simulink model "vehicle4"  (R2017a)
settings: Solver=VariableStepAuto  StartTime=0.0  StopTime=50  RelTol=1e-3
values from neighbouring files (symbols this model uses):
  Ts = 1    [dynorun.m]
undefined symbols (not defined in the file or in its folder): magnitude
undefined symbols (not defined in the file): containers
settings Model: Creator=tstef  LastModifiedBy=elts2

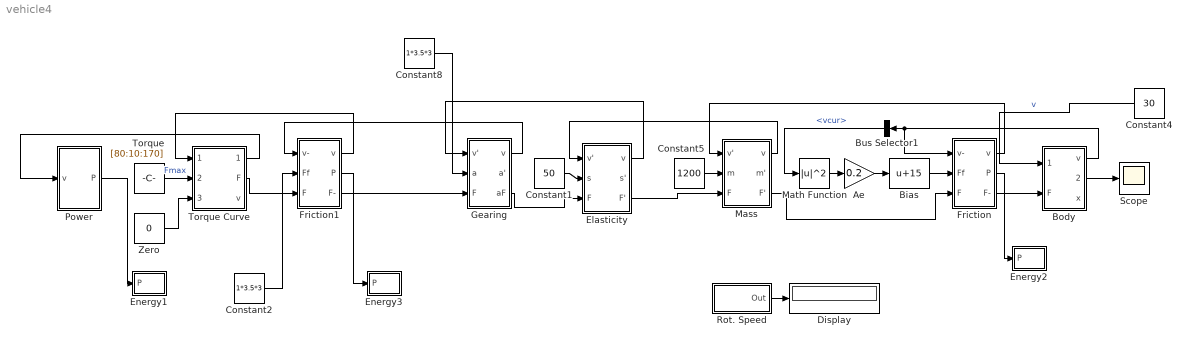
== system vehicle4 ==
  Ae : Gain  Gain=0.2
  Bias : Bias  Bias=15
  Body : Subsystem
  Bus Selector1 : BusSelector  OutputSignals=vcur
  Constant1 : Constant  Value=50
  Constant2 : Constant  Value=1*3.5*3
  Constant4 : Constant  Value=30
  Constant5 : Constant  Value=1200
  Constant8 : Constant  Value=1*3.5*3
  Display : Display
  Elasticity : Subsystem
  Energy1 : Subsystem
  Energy2 : Subsystem
  Energy3 : Subsystem
  Friction : Subsystem
  Friction1 : Subsystem
  Gearing : Subsystem
  Mass : Subsystem
  Math Function : Math  Operator=magnitude^2  SaturateOnIntegerOverflow=on
  Power : Subsystem
  Rot. Speed : Subsystem
  Scope : Scope
  Torque : Constant  Value=[80:10:170]
  Torque Curve : Subsystem
  Zero : Constant  Value=0
  wires:
  Constant8/1 -> Gearing/2(a)
  Gearing/3(aF) -> Elasticity/3(F)
  Mass/1(v) -> Elasticity/1(v')
  Mass/3(F') -> Friction/3(F)
  Friction/1(v) -> Mass/1(v')
  Constant5/1 -> Mass/2(m)
  Bias/1 -> Friction/2(Ff)
  Bus Selector1/1 -> Math Function/1  "<vcur>"
  Math Function/1 -> Ae/1
  Ae/1 -> Bias/1
  Gearing/1(v) -> Friction1/1(v-)
  Body/1(v) -> Bus Selector1/1, Friction/1(v-)
  Constant4/1 -> Body/1(vmax)  "v"
  Friction/3(F-) -> Body/2(F)
  Body/2(vcur) -> Scope/1
  Power/1(P) -> Energy1/1(P)
  Friction/2(P) -> Energy2/1(P)
  Elasticity/3(F') -> Mass/3(F)
  Elasticity/1(v) -> Gearing/1(v')
  Constant1/1 -> Elasticity/2(s)
  Rot. Speed/1(Out) -> Display/1
  Friction1/3(F-) -> Gearing/3(F)
  Friction1/1(v) -> Torque Curve/1(vreq)
  Constant2/1 -> Friction1/2(Ff)
  Friction1/2(P) -> Energy3/1(P)
  Torque Curve/2(F) -> Friction1/3(F)
  Torque Curve/1(vmax) -> Power/1(v)
  Torque/1 -> Torque Curve/2(Fmax)  "Fmax"
  Zero/1 -> Torque Curve/3(Fmin)

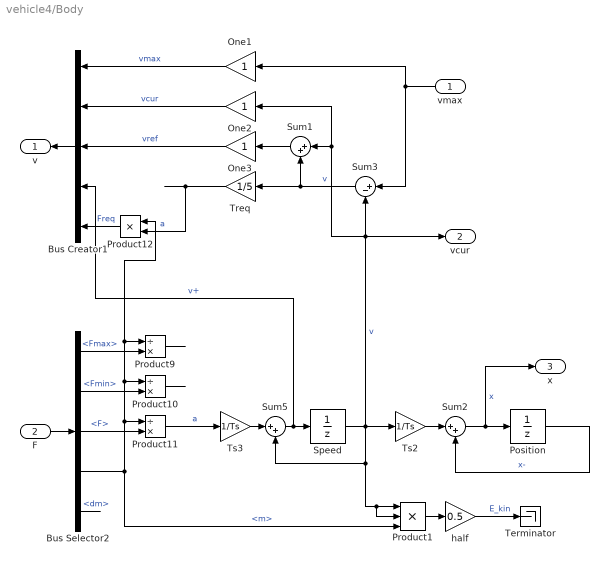
== system vehicle4/Body ==
  vmax : Inport  Unit=m/s
  F : Inport  Port=2
  Bus Creator1 : BusCreator  Inputs=5
  Bus Selector2 : BusSelector  OutputSignals=Fmax,Fmin,F,m,dm
  One1 : Gain
  One2 : Gain
  One3 : Gain
  Position : UnitDelay  InitialCondition=zeros(1,10)  SampleTime=Ts
  Product1 : Product  Inputs=***
  Product10 : Product  Inputs=/*
  Product11 : Product  Inputs=/*
  Product12 : Product
  Product9 : Product  Inputs=/*
  Speed : UnitDelay  InitialCondition=zeros(1,10)  SampleTime=Ts
  Sum1 : Sum  Inputs=|++
  Sum2 : Sum  Inputs=|++
  Sum3 : Sum  Inputs=|+-
  Sum5 : Sum  Inputs=|++
  Terminator : Terminator
  Treq : Gain  Gain=1/5
  Ts2 : Gain  Gain=1/Ts
  Ts3 : Gain  Gain=1/Ts
  half : Gain  Gain=0.5
  v : Outport
  vcur : Outport  Port=2
  x : Outport  Port=3
  wires:
  Treq/1 -> Product12/2  "a"
  Product11/1 -> Ts3/1  "a"
  One3/1 -> Bus Creator1/3  "vref"
  Product12/1 -> Bus Creator1/5  "Freq"
  Bus Selector2/5 -> ?  "<dm>"
  Sum1/1 -> One3/1
  One1/1 -> Bus Creator1/1  "vmax"
  F/1 -> Bus Selector2/1
  Bus Selector2/1 -> Product9/2  "<Fmax>"
  Bus Selector2/4 -> Product1/3, Product9/1, Product12/1, Product10/1, Product11/1  "<m>"
  Bus Selector2/3 -> Product11/2  "<F>"
  Bus Selector2/2 -> Product10/2  "<Fmin>"
  One2/1 -> Bus Creator1/2  "vcur"
  Speed/1 -> Ts2/1, vcur/1, Sum1/1, One2/1, Sum3/2, Sum5/2, Product1/2, Product1/1  "v"
  vmax/1 -> Sum3/1, One1/1
  Sum3/1 -> Sum1/2, Treq/1  "v"
  Sum5/1 -> Bus Creator1/4, Speed/1  "v+"
  Ts3/1 -> Sum5/1
  Product9/1 -> ?
  Product10/1 -> ?
  Bus Creator1/1 -> v/1
  Product1/1 -> half/1
  half/1 -> Terminator/1  "E_kin"
  Sum2/1 -> x/1, Position/1  "x"
  Position/1 -> Sum2/2  "x-"
  Ts2/1 -> Sum2/1

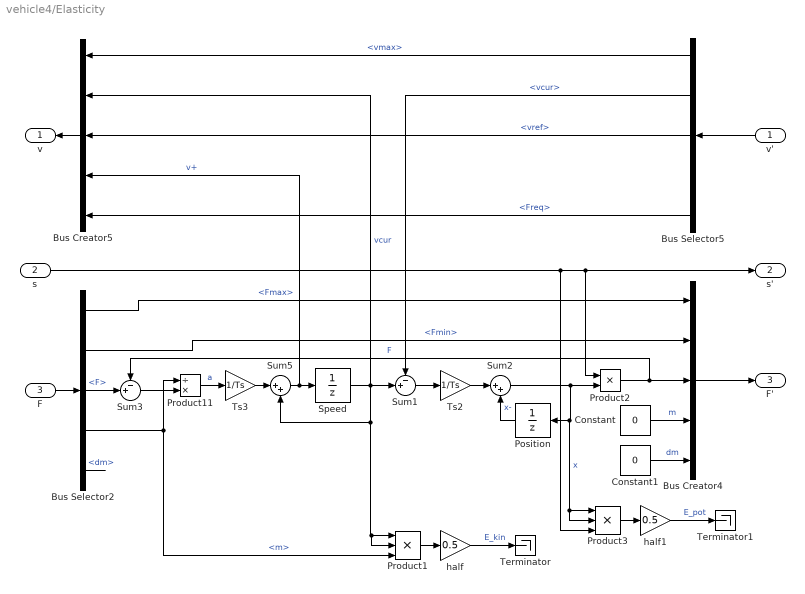
== system vehicle4/Elasticity ==
  v' : Inport
  s : Inport  Port=2
  F : Inport  Port=3
  Bus Creator4 : BusCreator  Inputs=5
  Bus Creator5 : BusCreator  Inputs=5
  Bus Selector2 : BusSelector  OutputSignals=Fmax,Fmin,F,m,dm
  Bus Selector5 : BusSelector  OutputSignals=vmax,vcur,vref,v+,Freq
  Constant : Constant  Value=0
  Constant1 : Constant  Value=0
  Position : UnitDelay  InitialCondition=zeros(1,10)  SampleTime=Ts
  Product1 : Product  Inputs=***
  Product11 : Product  Inputs=/*
  Product2 : Product  Inputs=**
  Product3 : Product  Inputs=***
  Speed : UnitDelay  InitialCondition=zeros(1,10)  SampleTime=Ts
  Sum1 : Sum  Inputs=-+|
  Sum2 : Sum  Inputs=|++
  Sum3 : Sum  Inputs=-+|
  Sum5 : Sum  Inputs=|++
  Terminator : Terminator
  Terminator1 : Terminator
  Ts2 : Gain  Gain=1/Ts
  Ts3 : Gain  Gain=1/Ts
  half : Gain  Gain=0.5
  half1 : Gain  Gain=0.5
  v : Outport
  s' : Outport  Port=2
  F' : Outport  Port=3
  wires:
  Bus Creator5/1 -> v/1
  v'/1 -> Bus Selector5/1
  Bus Selector5/2 -> Sum1/1  "<vcur>"
  Bus Selector5/1 -> Bus Creator5/1  "<vmax>"
  Bus Creator4/1 -> F'/1
  Bus Selector2/4 -> Product1/3, Product11/1  "<m>"
  Ts2/1 -> Sum2/1
  Speed/1 -> Bus Creator5/2, Sum1/2, Sum5/2, Product1/2, Product1/1  "vcur"
  Product11/1 -> Ts3/1  "a"
  Position/1 -> Sum2/2  "x-"
  Ts3/1 -> Sum5/1
  Product1/1 -> half/1
  Sum5/1 -> Bus Creator5/4, Speed/1  "v+"
  Sum2/1 -> Product2/2, Product3/2, Product3/1, Position/1  "x"
  Bus Selector2/3 -> Sum3/2  "<F>"
  F/1 -> Bus Selector2/1
  half/1 -> Terminator/1  "E_kin"
  Bus Selector2/5 -> ?  "<dm>"
  Sum1/1 -> Ts2/1
  Bus Selector5/3 -> Bus Creator5/3  "<vref>"
  Bus Selector5/5 -> Bus Creator5/5  "<Freq>"
  s/1 -> Product3/3, s'/1, Product2/1
  Product2/1 -> Sum3/1, Bus Creator4/3  "F"
  Bus Selector2/2 -> Bus Creator4/2  "<Fmin>"
  Bus Selector2/1 -> Bus Creator4/1  "<Fmax>"
  Constant/1 -> Bus Creator4/4  "m"
  Constant1/1 -> Bus Creator4/5  "dm"
  half1/1 -> Terminator1/1  "E_pot"
  Product3/1 -> half1/1
  Sum3/1 -> Product11/2

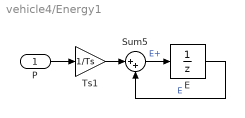
== system vehicle4/Energy1 ==
  P : Inport
  E : UnitDelay  InitialCondition=zeros(1,10)  SampleTime=Ts
  Sum5 : Sum  Inputs=|++
  Ts1 : Gain  Gain=1/Ts
  wires:
  E/1 -> Sum5/2  "E"
  Sum5/1 -> E/1  "E+"
  P/1 -> Ts1/1
  Ts1/1 -> Sum5/1

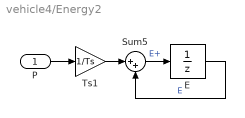
== system vehicle4/Energy2 ==
  P : Inport
  E : UnitDelay  InitialCondition=zeros(1,10)  SampleTime=Ts
  Sum5 : Sum  Inputs=|++
  Ts1 : Gain  Gain=1/Ts
  wires:
  P/1 -> Ts1/1
  Sum5/1 -> E/1  "E+"
  E/1 -> Sum5/2  "E"
  Ts1/1 -> Sum5/1

== system vehicle4/Energy3 ==
  P : Inport
  E : UnitDelay  InitialCondition=zeros(1,10)  SampleTime=Ts
  Sum5 : Sum  Inputs=|++
  Ts1 : Gain  Gain=1/Ts
  wires:
  Ts1/1 -> Sum5/1
  P/1 -> Ts1/1
  Sum5/1 -> E/1  "E+"
  E/1 -> Sum5/2  "E"

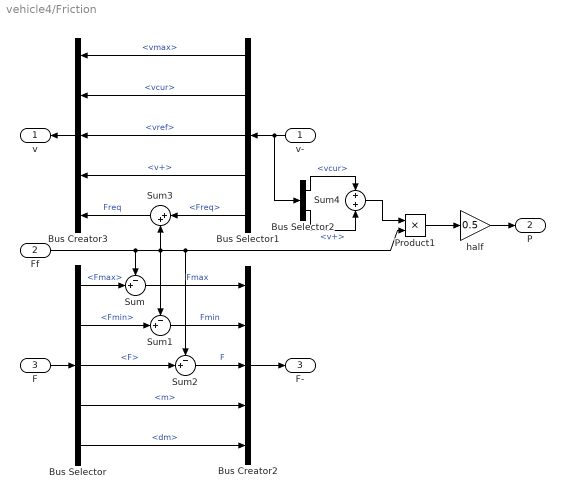
== system vehicle4/Friction ==
  v- : Inport
  Ff : Inport  Port=2
  F : Inport  Port=3
  Bus Creator2 : BusCreator  Inputs=5
  Bus Creator3 : BusCreator  Inputs=5
  Bus Selector : BusSelector  OutputSignals=Fmax,Fmin,F,m,dm
  Bus Selector1 : BusSelector  OutputSignals=vmax,vcur,vref,v+,Freq
  Bus Selector2 : BusSelector  OutputSignals=vcur,v+
  Product1 : Product
  Sum : Sum  Inputs=-+|
  Sum1 : Sum  Inputs=-+|
  Sum2 : Sum  Inputs=-+|
  Sum3 : Sum  Inputs=|++
  Sum4 : Sum
  half : Gain  Gain=0.5
  v : Outport
  P : Outport  Port=2
  F- : Outport  Port=3
  wires:
  F/1 -> Bus Selector/1
  Bus Creator3/1 -> v/1
  Bus Selector/5 -> Bus Creator2/5  "<dm>"
  Ff/1 -> Sum/1, Sum3/2, Sum1/1, Product1/2, Sum2/1
  Bus Creator2/1 -> F-/1
  Bus Selector1/1 -> Bus Creator3/1  "<vmax>"
  Bus Selector1/2 -> Bus Creator3/2  "<vcur>"
  Bus Selector1/3 -> Bus Creator3/3  "<vref>"
  Bus Selector1/4 -> Bus Creator3/4  "<v+>"
  Bus Selector/4 -> Bus Creator2/4  "<m>"
  Bus Selector/3 -> Sum2/2  "<F>"
  Bus Selector/2 -> Sum1/2  "<Fmin>"
  Bus Selector/1 -> Sum/2  "<Fmax>"
  Sum/1 -> Bus Creator2/1  "Fmax"
  Sum1/1 -> Bus Creator2/2  "Fmin"
  Sum2/1 -> Bus Creator2/3  "F"
  Bus Selector1/5 -> Sum3/1  "<Freq>"
  Sum3/1 -> Bus Creator3/5  "Freq"
  Product1/1 -> half/1
  Sum4/1 -> Product1/1
  v-/1 -> Bus Selector2/1, Bus Selector1/1
  half/1 -> P/1
  Bus Selector2/2 -> Sum4/2  "<v+>"
  Bus Selector2/1 -> Sum4/1  "<vcur>"

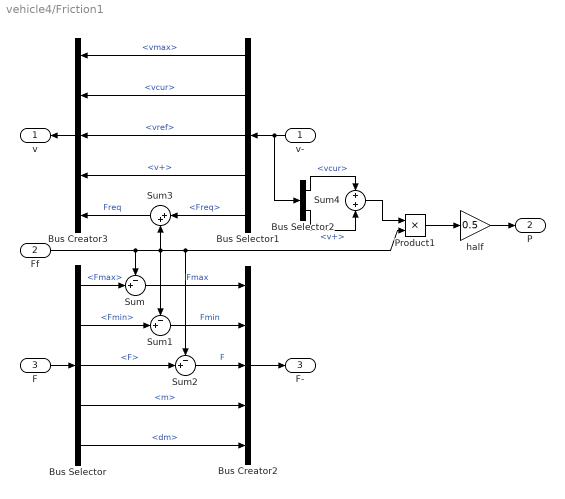
== system vehicle4/Friction1 ==
  v- : Inport
  Ff : Inport  Port=2
  F : Inport  Port=3
  Bus Creator2 : BusCreator  Inputs=5
  Bus Creator3 : BusCreator  Inputs=5
  Bus Selector : BusSelector  OutputSignals=Fmax,Fmin,F,m,dm
  Bus Selector1 : BusSelector  OutputSignals=vmax,vcur,vref,v+,Freq
  Bus Selector2 : BusSelector  OutputSignals=vcur,v+
  Product1 : Product
  Sum : Sum  Inputs=-+|
  Sum1 : Sum  Inputs=-+|
  Sum2 : Sum  Inputs=-+|
  Sum3 : Sum  Inputs=|++
  Sum4 : Sum
  half : Gain  Gain=0.5
  v : Outport
  P : Outport  Port=2
  F- : Outport  Port=3
  wires:
  Bus Selector2/1 -> Sum4/1  "<vcur>"
  Bus Selector2/2 -> Sum4/2  "<v+>"
  half/1 -> P/1
  v-/1 -> Bus Selector1/1, Bus Selector2/1
  Sum4/1 -> Product1/1
  Product1/1 -> half/1
  Sum3/1 -> Bus Creator3/5  "Freq"
  Bus Selector1/5 -> Sum3/1  "<Freq>"
  Sum2/1 -> Bus Creator2/3  "F"
  Sum1/1 -> Bus Creator2/2  "Fmin"
  Sum/1 -> Bus Creator2/1  "Fmax"
  Bus Selector/1 -> Sum/2  "<Fmax>"
  Bus Selector/2 -> Sum1/2  "<Fmin>"
  Bus Selector/3 -> Sum2/2  "<F>"
  Bus Selector/4 -> Bus Creator2/4  "<m>"
  Bus Selector1/4 -> Bus Creator3/4  "<v+>"
  Bus Selector1/3 -> Bus Creator3/3  "<vref>"
  Bus Selector1/2 -> Bus Creator3/2  "<vcur>"
  Bus Selector1/1 -> Bus Creator3/1  "<vmax>"
  Bus Creator2/1 -> F-/1
  Ff/1 -> Sum2/1, Product1/2, Sum1/1, Sum3/2, Sum/1
  Bus Selector/5 -> Bus Creator2/5  "<dm>"
  Bus Creator3/1 -> v/1
  F/1 -> Bus Selector/1

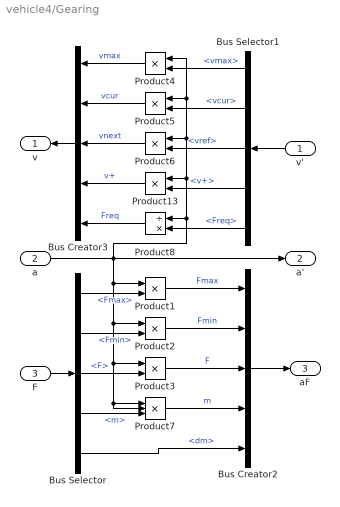
== system vehicle4/Gearing ==
  v' : Inport
  a : Inport  Port=2
  F : Inport  Port=3
  Bus Creator2 : BusCreator  Inputs=5
  Bus Creator3 : BusCreator  Inputs=5
  Bus Selector : BusSelector  OutputSignals=Fmax,Fmin,F,m,dm
  Bus Selector1 : BusSelector  OutputSignals=vmax,vcur,vref,v+,Freq
  Product{1..6,13} (7 alike) : Product
  Product7 : Product  Inputs=***
  Product8 : Product  Inputs=/*
  v : Outport
  a' : Outport  Port=2
  aF : Outport  Port=3
  wires:
  Bus Creator2/1 -> aF/1
  Product5/1 -> Bus Creator3/2  "vcur"
  Bus Selector1/5 -> Product8/2  "<Freq>"
  Product3/1 -> Bus Creator2/3  "F"
  Product4/1 -> Bus Creator3/1  "vmax"
  Product7/1 -> Bus Creator2/4  "m"
  a/1 -> Product13/1, Product4/1, Product5/1, Product6/1, Product8/1, a'/1, Product7/1, Product7/2, Product3/1, Product2/1, Product1/1
  Bus Selector/4 -> Product7/3  "<m>"
  Bus Selector/1 -> Product1/2  "<Fmax>"
  Bus Selector/3 -> Product3/2  "<F>"
  Bus Selector/5 -> Bus Creator2/5  "<dm>"
  Bus Selector/2 -> Product2/2  "<Fmin>"
  Bus Creator3/1 -> v/1
  Product1/1 -> Bus Creator2/1  "Fmax"
  Product8/1 -> Bus Creator3/5  "Freq"
  Bus Selector1/3 -> Product6/2  "<vref>"
  F/1 -> Bus Selector/1
  Bus Selector1/2 -> Product5/2  "<vcur>"
  Bus Selector1/1 -> Product4/2  "<vmax>"
  Product6/1 -> Bus Creator3/3  "vnext"
  Product2/1 -> Bus Creator2/2  "Fmin"
  Product13/1 -> Bus Creator3/4  "v+"
  Bus Selector1/4 -> Product13/2  "<v+>"
  v'/1 -> Bus Selector1/1

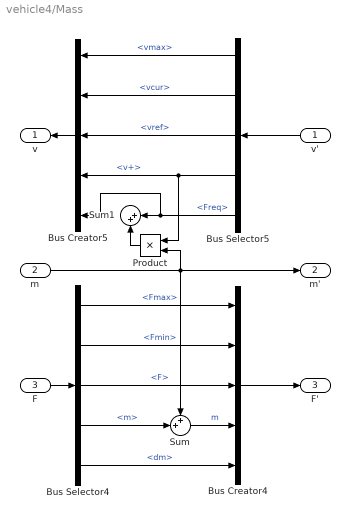
== system vehicle4/Mass ==
  v' : Inport
  m : Inport  Port=2
  F : Inport  Port=3
  Bus Creator4 : BusCreator  Inputs=5
  Bus Creator5 : BusCreator  Inputs=5
  Bus Selector4 : BusSelector  OutputSignals=Fmax,Fmin,F,m,dm
  Bus Selector5 : BusSelector  OutputSignals=vmax,vcur,vref,v+,Freq
  Product : Product
  Sum : Sum  Inputs=++|
  Sum1 : Sum  Inputs=|++
  v : Outport
  m' : Outport  Port=2
  F' : Outport  Port=3
  wires:
  Bus Selector4/5 -> Bus Creator4/5  "<dm>"
  Bus Creator4/1 -> F'/1
  Bus Selector4/1 -> Bus Creator4/1  "<Fmax>"
  Sum/1 -> Bus Creator4/4  "m"
  Bus Selector4/3 -> Bus Creator4/3  "<F>"
  Bus Selector5/3 -> Bus Creator5/3  "<vref>"
  Bus Selector5/4 -> Product/1, Bus Creator5/4  "<v+>"
  Bus Selector5/1 -> Bus Creator5/1  "<vmax>"
  Bus Selector5/5 -> Bus Creator5/5, Sum1/1  "<Freq>"
  Bus Selector5/2 -> Bus Creator5/2  "<vcur>"
  Bus Selector4/4 -> Sum/2  "<m>"
  v'/1 -> Bus Selector5/1
  Bus Selector4/2 -> Bus Creator4/2  "<Fmin>"
  F/1 -> Bus Selector4/1
  Bus Creator5/1 -> v/1
  m/1 -> Product/2, Sum/1, m'/1
  Product/1 -> Sum1/2

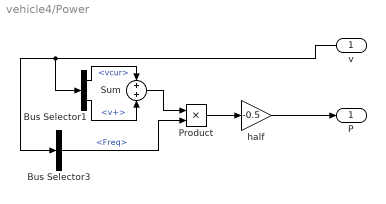
== system vehicle4/Power ==
  v : Inport
  Bus Selector1 : BusSelector  OutputSignals=vcur,v+
  Bus Selector3 : BusSelector  OutputSignals=Freq
  Product : Product
  Sum : Sum
  half : Gain  Gain=-0.5
  P : Outport
  wires:
  v/1 -> Bus Selector1/1, Bus Selector3/1
  Bus Selector1/1 -> Sum/1  "<vcur>"
  Product/1 -> half/1
  half/1 -> P/1
  Bus Selector1/2 -> Sum/2  "<v+>"
  Sum/1 -> Product/1
  Bus Selector3/1 -> Product/2  "<Freq>"

== system vehicle4/Rot. Speed ==
  Constant : Subsystem  mask(Constant value with units){Value=10, unitstr=rpm, unitmap=containers.Map({'rad/s','Hz','rpm','hrpm','krpm'},[1 2*pi 2*pi/60 2*pi/60*100 2*pi/60*1000])}
      mask prompts: Value "Simulink:blkprm_prompts:ConstConstValue"; unitmap "Unit map:"
      mask help:
      | This is a generic block for a value with units.
      |
      | The units can be configured with the field unitmap.
      mask TypeOptions Value: Constant/Value
      mask TypeOptions unitstr: rad/s | rpm | hrpm | krpm | Hz
      mask Display: disp(string(Value))
  Out : Outport
  wires:
  Constant/1(Out) -> Out/1

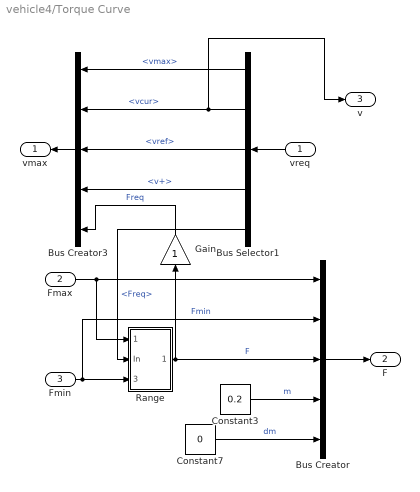
== system vehicle4/Torque Curve ==
  vreq : Inport
  Fmax : Inport  Port=2
  Fmin : Inport  Port=3
  Bus Creator : BusCreator  Inputs=5
  Bus Creator3 : BusCreator  Inputs=5
  Bus Selector1 : BusSelector  OutputSignals=vmax,vcur,vref,v+,Freq
  Constant3 : Constant  Value=0.2
  Constant7 : Constant  Value=0
  Gain : Gain
  Range : Subsystem
  vmax : Outport
  F : Outport  Port=2
  v : Outport  Port=3
  wires:
  Bus Creator/1 -> F/1
  Fmax/1 -> Range/1(Max), Bus Creator/1
  Constant3/1 -> Bus Creator/4  "m"
  Constant7/1 -> Bus Creator/5  "dm"
  Fmin/1 -> Bus Creator/2, Range/3(Min)  "Fmin"
  Bus Selector1/2 -> v/1, Bus Creator3/2  "<vcur>"
  Bus Creator3/1 -> vmax/1
  vreq/1 -> Bus Selector1/1
  Bus Selector1/3 -> Bus Creator3/3  "<vref>"
  Bus Selector1/1 -> Bus Creator3/1  "<vmax>"
  Bus Selector1/4 -> Bus Creator3/4  "<v+>"
  Bus Selector1/5 -> Range/2(In)  "<Freq>"
  Range/1(Out) -> Bus Creator/3, Gain/1  "F"
  Gain/1 -> Bus Creator3/5  "Freq"

== system vehicle4/Rot. Speed/Constant ==
  Constant : Constant  Value=Value
  Unit : Gain  Gain=unitmap(unitstr)
  Out : Outport
  wires:
  Unit/1 -> Out/1
  Constant/1 -> Unit/1

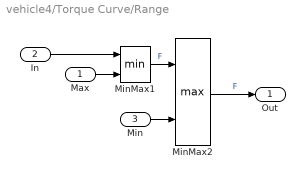
== system vehicle4/Torque Curve/Range ==
  Max : Inport
  In : Inport  Port=2
  Min : Inport  Port=3
  MinMax1 : MinMax  Inputs=2
  MinMax2 : MinMax  Function=max  Inputs=2
  Out : Outport
  wires:
  Max/1 -> MinMax1/2
  Min/1 -> MinMax2/2
  MinMax2/1 -> Out/1  "F"
  In/1 -> MinMax1/1
  MinMax1/1 -> MinMax2/1  "F"
